simulink model "untitled"  (R2020b)
settings: Solver=VariableStepAuto  StartTime=0.0  StopTime=10.0  RelTol=1e-3
settings Model: Creator=macbook  LastModifiedBy=macbook

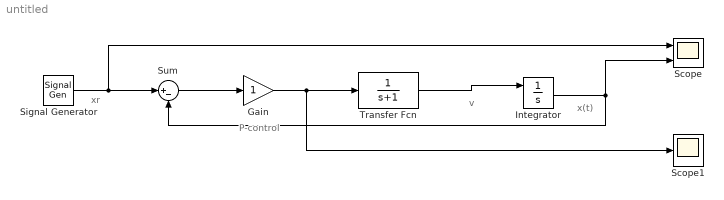
== system untitled ==
  note: xr
  note: x(t)
  note: P-control
  note: v
  Gain : Gain
  Integrator : Integrator  InitialConditionSource=external  AbsoluteTolerance=0.3
  Scope : Scope  NumInputPorts=2
  Scope1 : Scope
  Signal Generator : SignalGenerator  Units=rad/sec
  Sum : Sum  Inputs=|+-
  Transfer Fcn : TransferFcn  Numerator=1  Denominator=[1 1]  AbsoluteTolerance=0.1
  wires:
  Sum/1 -> Gain/1
  Gain/1 -> Scope1/1, Transfer Fcn/1
  Transfer Fcn/1 -> Integrator/1
  Integrator/1 -> Scope/2, Sum/2
  Signal Generator/1 -> Scope/1, Sum/1
